simulink model "VSG_control_model"  (R2022b)
settings: Solver=ode23t  StartTime=0.0  StopTime=0.2  FixedStep=1e-6  RelTol=1e-3
InitFcn:
  | f = 20e3;%视频是20e3
  | Ts = 1/f;
  | 
  | %Vdc = 800;L1 = 3.2e-3;C = 10e-6;R = 0.5;L2 = 800e-6;RC = 0.001;
  | 
  | fn = 50; %工频
  | Ub = 6000;
  | Sb = 800e3;%容量800kVA
  | Ib = Sb/(sqrt(3)*Ub);
  | w0 = 2*pi*fn;
  | J = 3.36; %转动惯量
  | D = 3.24e4/w0; %阻尼系数
  | kf = 0.95e4/w0; %一次调频系数
  | kq = (2500*6000)/(800e3*sqrt(3)); %无功调压系数
  | ki = 0.5*sqrt(3)*Sb/Ub;%无功调节积分控制器
  | 
  | L=3e-3;%滤波电感
  | Rf = 0.05;%电感电阻
  | Cf = 35e-6;%滤波电容
  | R = 0.5;%无源阻尼
  | Un = 380;%网侧电压给定
undefined symbols (not defined in the file): Simulation
libraries: spsSeriesRLCBranchLib x11, spsMosfetLib x6, spsThreePhaseVIMeasurementLib x3, spsGroundLib x2, spsThreePhaseSeriesRLCBranchLib x1, eePowerMeasurement x1, dspstat3 x1, simulink x1, spsThreePhaseProgrammableVoltageSourceLib x1, spsDCVoltageSourceLib x1, sps_lib x1, spsThreePhaseSeriesRLCLoadLib x1
settings Model: Creator=Li  LastModifiedBy=Li
settings DataIOCC: ReturnWorkspaceOutputs=off

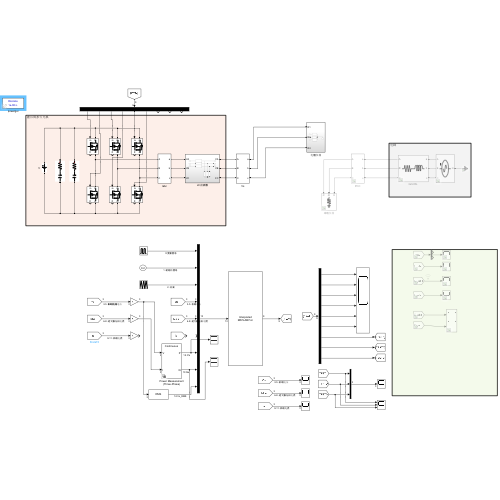
[thumbnail: Simulink's stored preview of the top-level diagram]
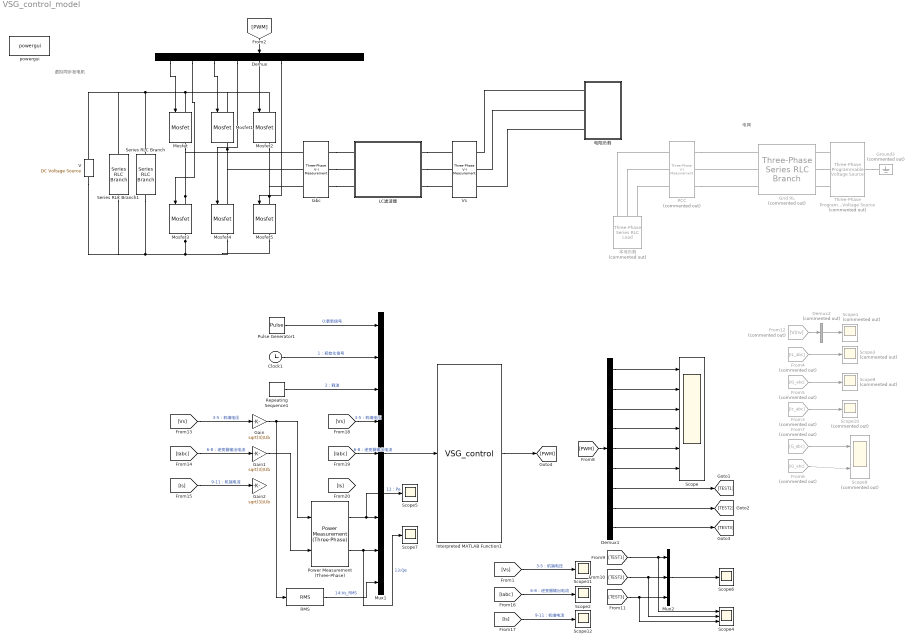
== system VSG_control_model ==
  note: 电网
  note: 虚拟同步发电机
  Clock1 : Clock
  Demux : Demux  Outputs=9
  Demux1 : Demux  Outputs=9
  Demux2 : Demux  Commented=on  Outputs=3
  From12 : From  Commented=on  GotoTag=Vinv  TagVisibility=global
  From3 : From  Commented=on  GotoTag=Ic_abc  TagVisibility=global
  From4 : From  Commented=on  GotoTag=IL_abc  TagVisibility=global
  From5 : From  Commented=on  GotoTag=IG_abc  TagVisibility=global
  From6 : From  Commented=on  GotoTag=IG_abc  TagVisibility=global
  From7 : From  Commented=on  GotoTag=G_abc  TagVisibility=global
  Gain : Gain  Gain=sqrt(3)/Ub
  Gain1 : Gain  Gain=sqrt(3)/Ub
  Gain2 : Gain  Gain=sqrt(3)/Ub
  Grid RL : spsThreePhaseSeriesRLCBranchLib/Three-Phase Series RLC Branch  Commented=on  LConnTagsString=A|B|C  RConnTagsString=A|B|C  BranchType=RL  Resistance=0.06  Inductance=1.35e-3  Capacitance=1e-6  Measurements=None
  Ground3 : spsGroundLib/Ground  Commented=on  LConnTagsString=a
  Iabc : spsThreePhaseVIMeasurementLib/Three-Phase V-I Measurement  VoltageMeasurement=no  SetLabelV=on  LabelV=Vs  Vpu=off  VpuLL=off  CurrentMeasurement=yes  SetLabelI=on  LabelI=Iabc  Ipu=off  Pbase=100e6  Vbase=500e3  OutputType=Complex  PhasorSimulation=off  PSBequivalent=0
  Interpreted MATLAB Function1 : MATLABFcn  MATLABFcn=VSG_control  OutputDimensions=9
  LC滤波器 : Subsystem
  Mosfet{,1..5} (6 alike) : spsMosfetLib/Mosfet  Ron=0.1  Lon=0  Rd=0.01  Vfd=0  IC=0  Rs=1e5  Cs=inf  Measurements=on
  Mux1 : Mux  Inputs=9
  Mux2 : Mux  Inputs=3
  PCC : spsThreePhaseVIMeasurementLib/Three-Phase V-I Measurement  Commented=on  VoltageMeasurement=phase-to-ground  SetLabelV=on  LabelV=Vg  Vpu=off  VpuLL=off  CurrentMeasurement=yes  SetLabelI=on  LabelI=Ig  Ipu=off  Pbase=100e6  Vbase=500e3  OutputType=Complex  PhasorSimulation=off  PSBequivalent=0
  Power Measurement (Three-Phase) : eePowerMeasurement/Power Measurement (Three-Phase)  LabelModeActiveChoice=Continuous  F=50  K=[1]  Seq=Positive  Ts=0
  Pulse Generator1 : DiscretePulseGenerator  PulseType=Time based  Period=Ts  PulseWidth=50
  RMS : dspstat3/RMS  run=off  directionMode=Each column  dimension=1  InputProcessing=Columns as channels (frame based)  reset_popup=None
  Repeating Sequence1 : simulink/Sources/Repeating Sequence  rep_seq_t=[0 Ts/2 Ts]  rep_seq_y=[0 1 0]
  Scope : Scope  NumInputPorts=6
  Scope{1,3,8,10} (4 alike) : Scope  Commented=on
  Scope{2,5..7,11..12} (6 alike) : Scope
  Scope4 : Scope  NumInputPorts=3
  Scope9 : Scope  Commented=on  NumInputPorts=2
  Series RLC Branch : spsSeriesRLCBranchLib/Series RLC Branch  LConnTagsString=__new0  RConnTagsString=__new0  BranchType=RC  Resistance=1e-9  Inductance=1e-3  SetiL0=off  InitialCurrent=0  Capacitance=660e-6  Setx0=off  InitialVoltage=0  Measurements=None
  Series RLC Branch1 : spsSeriesRLCBranchLib/Series RLC Branch  LConnTagsString=__new0  RConnTagsString=__new0  BranchType=RC  Resistance=1e-9  Inductance=1e-3  SetiL0=off  InitialCurrent=0  Capacitance=23.5e-6  Setx0=off  InitialVoltage=0  Measurements=None
  Three-Phase Programmable Voltage Source : spsThreePhaseProgrammableVoltageSourceLib/Three-Phase Programmable Voltage Source  Commented=on  PositiveSequence="[380  0 50]"  VariationEntity=Frequency  VariationType=Table of time-amplitude pairs  VariationTypeAlt=Step  VariationStep=-0.2  VariationRate=10  VariationMagnitude=0.3  VariationFrequency=2  VariationTiming=[1 2]  VariationPhaseA=off  Amplitudes=[1 0.8 1.2 1.0]  TimeValues=[0 0.1 0.15 0.2]  HarmonicGeneration=off  HarmonicA=[3 0.2 -25 0]  HarmonicB=[2 0.15 35 2]  Timing="[0.05  3]"  BusType=swing  Pref=0  Qref=0  Qmin=-inf  Qmax=inf
  V : spsDCVoltageSourceLib/DC Voltage Source  Amplitude=1000  Measurements=Voltage
  Vs : spsThreePhaseVIMeasurementLib/Three-Phase V-I Measurement  VoltageMeasurement=phase-to-ground  SetLabelV=on  LabelV=Vs  Vpu=off  VpuLL=off  CurrentMeasurement=yes  SetLabelI=on  LabelI=Is  Ipu=off  Pbase=100e6  Vbase=500e3  OutputType=Complex  PhasorSimulation=off  PSBequivalent=0
  powergui : sps_lib/powergui  Priority=1  SimulationMode=Discrete  SampleTime=1e-6  frequency=60  Iterations=50  frequencyindice=0  Pbase=100e6  ErrMax=1e-4  UnitsV=kV  UnitsW=MW  buscounter=0  FunctionMessages=off  echomessages=off  EnableUseOfTLC=off  CurrentSourceSwitches=off  DisableSnubberDevices=off  DisableRonSwitches=off  DisableVfSwitches=off  DisplayEquations=off  AutomaticDiscreteSolvers=off  SolverType=Tustin/Backward Euler (TBE)  Interpol=off  ExternalGateDelay=off  methode=off  Ts=100  x0status=blocks  SPID=on  SwTol=0  HookPort=off  NonlinearTolerance=1e-4  nMaxIteration=100  ContinueOnMaxIteration=off  RestoreLinks=warning  ResistiveCurrentMeasurement=off  Frange=[0:2:500]  Ylog=off  Xlog=on  ShowGrid=off  save=off  variable=ZData  structure=0  ZoomFFT=off  StartTime=0.0  cycles=1  DisplayStyle=1  fundamental=60  FreqAxis=off  MaxFrequency=1000  frequencyindicesteady=1  RmsSteady=1  display=off
  本地负载 : spsThreePhaseSeriesRLCLoadLib/Three-Phase Series RLC Load  Commented=on  LConnTagsString=A|B|C  Configuration=Y (grounded)  NominalVoltage=380  Vabc=[1e3 1e3 1e3]  Vabcp=[1e3 1e3 1e3]  NominalFrequency=50  UnbalancedPower=off  ActivePower=120e3  InductivePower=0  CapacitivePower=0  Pabc=[10e3 9e3 11e3]  QLabc=[100 90 110]  QCabc=[100 90 110]  Pabcp=[10e3 9e3 11e3]  QLabcp=[100 90 110]  QCabcp=[100 90 110]  Measurements=None  LoadType=constant Z
  电阻负载 : Subsystem
  wires:
  [PWM] -> Demux/1
  Demux/1 -> Mosfet/1
  Demux/2 -> Mosfet3/1
  Demux/3 -> Mosfet1/1
  Demux/4 -> Mosfet4/1
  Demux/5 -> Mosfet2/1
  Demux/6 -> Mosfet5/1
  Demux1/1 -> Scope/1
  Demux1/2 -> Scope/2
  Demux1/3 -> Scope/3
  Demux1/4 -> Scope/4
  Demux1/5 -> Scope/5
  Demux1/6 -> Scope/6
  Demux1/7 -> [TEST1]
  Demux1/9 -> [TEST3]
  Mux2/1 -> Scope6/1
  From4/1 -> Scope3/1
  From5/1 -> Scope8/1
  From7/1 -> Scope9/1
  From6/1 -> Scope9/2
  From3/1 -> Scope10/1
  [PWM] -> Demux1/1
  Demux1/8 -> [TEST2]
  [TEST1] -> Scope4/1, Mux2/1
  [TEST2] -> Scope4/2, Mux2/2
  [TEST3] -> Scope4/3, Mux2/3
  From12/1 -> Demux2/1
  Demux2/2 -> Scope1/1
  [Vs] -> Gain/1  "3-5：机端电压"
  [Iabc] -> Gain1/1  "6-8：逆变器输出电流"
  Mux1/1 -> Interpreted MATLAB Function1/1
  Power Measurement (Three-Phase)/1 -> Scope5/1, Mux1/7  "12：Pe"
  Power Measurement (Three-Phase)/2 -> Scope7/1, Mux1/8  "13:Qe"
  Interpreted MATLAB Function1/1 -> [PWM]
  Pulse Generator1/1 -> Mux1/1  "0:更新信号"
  Clock1/1 -> Mux1/2  "1：初始化信号"
  Repeating Sequence1/1 -> Mux1/3  "2：载波"
  [Is] -> Gain2/1  "9-11：机端电流"
  Gain/1 -> RMS/1, Power Measurement (Three-Phase)/1
  Gain1/1 -> Power Measurement (Three-Phase)/2
  RMS/1 -> Mux1/9  "14:Vs_RMS"
  [Vs] -> Scope11/1  "3-5：机端电压"
  [Iabc] -> Scope2/1  "6-8：逆变器输出电流"
  [Is] -> Scope12/1  "9-11：机端电流"
  [Vs] -> Mux1/4  "3-5：机端电压"
  [Iabc] -> Mux1/5  "6-8：逆变器输出电流"
  connections:
  Series RLC Branch/LConn1 -- V/RConn1 -- Series RLC Branch1/LConn1 -- Mosfet2/LConn1 -- Mosfet1/LConn1 -- Mosfet/LConn1
  Mosfet1/RConn1 -- Iabc/LConn2 -- Mosfet4/LConn1
  Mosfet3/LConn1 -- Iabc/LConn1 -- Mosfet/RConn1
  Mosfet5/LConn1 -- Iabc/LConn3 -- Mosfet2/RConn1
  Mosfet3/RConn1 -- V/LConn1 -- Series RLC Branch1/RConn1 -- Series RLC Branch/RConn1 -- Mosfet5/RConn1 -- Mosfet4/RConn1
  电阻负载/LConn1 -- Vs/RConn1
  电阻负载/LConn2 -- Vs/RConn2
  本地负载/LConn3 -- PCC/LConn3
  PCC/RConn1 -- Grid RL/LConn1
  Grid RL/LConn2 -- PCC/RConn2
  PCC/RConn3 -- Grid RL/LConn3
  Three-Phase Programmable Voltage Source/RConn1 -- Grid RL/RConn1
  Grid RL/RConn2 -- Three-Phase Programmable Voltage Source/RConn2
  Three-Phase Programmable Voltage Source/RConn3 -- Grid RL/RConn3
  Three-Phase Programmable Voltage Source/LConn1 -- Ground3/LConn1
  LC滤波器/RConn1 -- Vs/LConn1
  LC滤波器/RConn2 -- Vs/LConn2
  LC滤波器/RConn3 -- Vs/LConn3
  Iabc/RConn1 -- LC滤波器/LConn1
  Iabc/RConn2 -- LC滤波器/LConn2
  Iabc/RConn3 -- LC滤波器/LConn3
  电阻负载/LConn3 -- Vs/RConn3
  本地负载/LConn2 -- PCC/LConn2
  本地负载/LConn1 -- PCC/LConn1

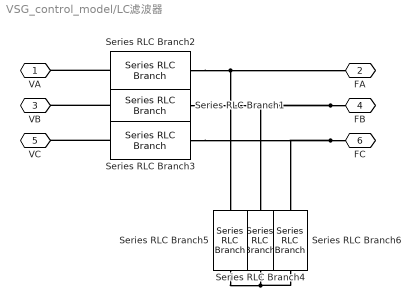
== system VSG_control_model/LC滤波器 ==
  Series RLC Branch1 : spsSeriesRLCBranchLib/Series RLC Branch  LConnTagsString=__new0  RConnTagsString=__new0  BranchType=RL  Resistance=Rf  Inductance=L  SetiL0=off  InitialCurrent=0  Capacitance=1e-3  Setx0=off  InitialVoltage=0  Measurements=None
  Series RLC Branch2 : spsSeriesRLCBranchLib/Series RLC Branch  LConnTagsString=__new0  RConnTagsString=__new0  BranchType=RL  Resistance=Rf  Inductance=L  SetiL0=off  InitialCurrent=0  Capacitance=1e-3  Setx0=off  InitialVoltage=0  Measurements=None
  Series RLC Branch3 : spsSeriesRLCBranchLib/Series RLC Branch  LConnTagsString=__new0  RConnTagsString=__new0  BranchType=RL  Resistance=Rf  Inductance=L  SetiL0=off  InitialCurrent=0  Capacitance=1e-3  Setx0=off  InitialVoltage=0  Measurements=None
  Series RLC Branch4 : spsSeriesRLCBranchLib/Series RLC Branch  LConnTagsString=__new0  RConnTagsString=__new0  BranchType=RC  Resistance=R  Inductance=Simulation.Inverter.Params.L1  SetiL0=off  InitialCurrent=0  Capacitance=Cf  Setx0=off  InitialVoltage=0  Measurements=None
  Series RLC Branch5 : spsSeriesRLCBranchLib/Series RLC Branch  LConnTagsString=__new0  RConnTagsString=__new0  BranchType=RC  Resistance=R  Inductance=Simulation.Inverter.Params.L1  SetiL0=off  InitialCurrent=0  Capacitance=Cf  Setx0=off  InitialVoltage=0  Measurements=None
  Series RLC Branch6 : spsSeriesRLCBranchLib/Series RLC Branch  LConnTagsString=__new0  RConnTagsString=__new0  BranchType=RC  Resistance=R  Inductance=Simulation.Inverter.Params.L1  SetiL0=off  InitialCurrent=0  Capacitance=Cf  Setx0=off  InitialVoltage=0  Measurements=None
  VA : PMIOPort  Side=Left
  FA : PMIOPort  Port=2  Side=Right
  VB : PMIOPort  Port=3  Side=Left
  FB : PMIOPort  Port=4  Side=Right
  VC : PMIOPort  Port=5  Side=Left
  FC : PMIOPort  Port=6  Side=Right
  connections:
  FC/RConn1 -- Series RLC Branch6/LConn1 -- Series RLC Branch3/RConn1
  Series RLC Branch5/RConn1 -- Series RLC Branch6/RConn1 -- Series RLC Branch4/RConn1
  Series RLC Branch2/RConn1 -- Series RLC Branch5/LConn1 -- FA/RConn1
  FB/RConn1 -- Series RLC Branch4/LConn1 -- Series RLC Branch1/RConn1
  Series RLC Branch1/LConn1 -- VB/RConn1
  Series RLC Branch3/LConn1 -- VC/RConn1
  Series RLC Branch2/LConn1 -- VA/RConn1

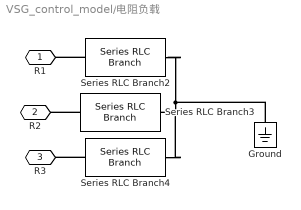
== system VSG_control_model/电阻负载 ==
  Ground : spsGroundLib/Ground  LConnTagsString=a
  Series RLC Branch2 : spsSeriesRLCBranchLib/Series RLC Branch  LConnTagsString=__new0  RConnTagsString=__new0  BranchType=R  Resistance=1  Inductance=L  SetiL0=off  InitialCurrent=0  Capacitance=1e-3  Setx0=off  InitialVoltage=0  Measurements=None
  Series RLC Branch3 : spsSeriesRLCBranchLib/Series RLC Branch  LConnTagsString=__new0  RConnTagsString=__new0  BranchType=R  Resistance=1  Inductance=L  SetiL0=off  InitialCurrent=0  Capacitance=1e-3  Setx0=off  InitialVoltage=0  Measurements=None
  Series RLC Branch4 : spsSeriesRLCBranchLib/Series RLC Branch  LConnTagsString=__new0  RConnTagsString=__new0  BranchType=R  Resistance=1  Inductance=L  SetiL0=off  InitialCurrent=0  Capacitance=1e-3  Setx0=off  InitialVoltage=0  Measurements=None
  R1 : PMIOPort  Side=Left
  R2 : PMIOPort  Port=2  Side=Left
  R3 : PMIOPort  Port=3  Side=Left
  connections:
  Series RLC Branch2/RConn1 -- Series RLC Branch4/RConn1 -- Series RLC Branch3/RConn1 -- Ground/LConn1
  Series RLC Branch4/LConn1 -- R3/RConn1
  Series RLC Branch2/LConn1 -- R1/RConn1
  Series RLC Branch3/LConn1 -- R2/RConn1
